simulink model "gm_sampleModel1630_sub"  (R2023a)
settings: Solver=VariableStepAuto  StartTime=0.0  StopTime=10.0  RelTol=1e-3
settings Model: Creator=user1  LastModifiedBy=user1
settings OptimizationCC: BlockReduction=off  ConditionallyExecuteInputs=off
settings DebuggingCC: InheritedTsInSrcMsg=none

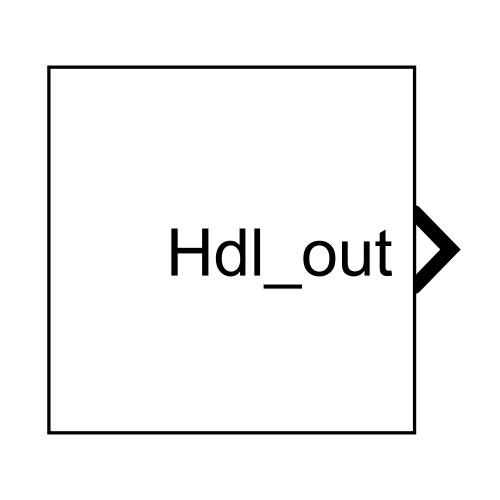
[thumbnail: Simulink's stored preview of the top-level diagram]
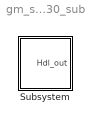
== system gm_sampleModel1630_sub ==
  Subsystem : Subsystem

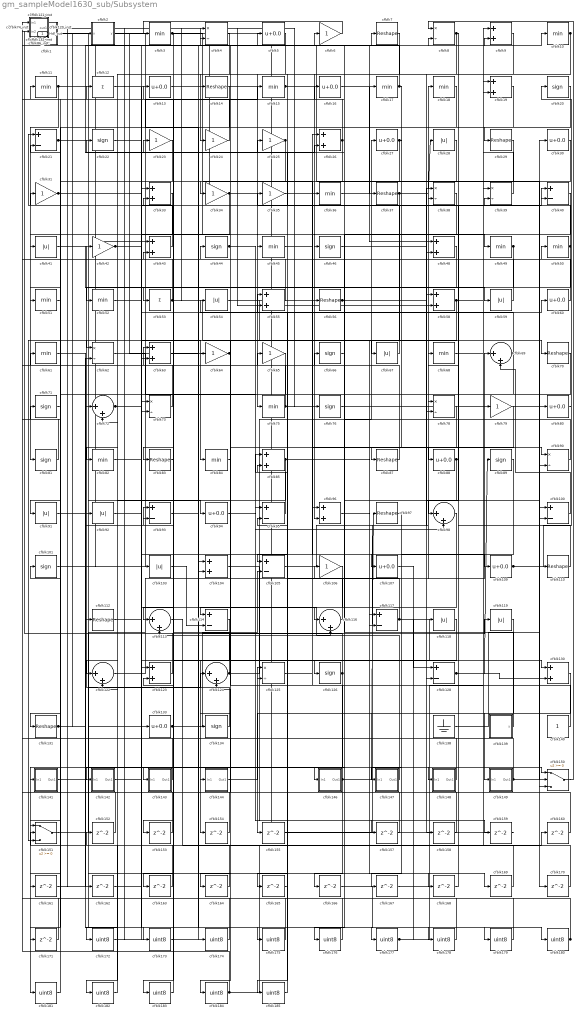
== system gm_sampleModel1630_sub/Subsystem ==
  cfblk1 : Subsystem  mask(Compare To Zero){relop=<=, OutDataTypeStr=uint8, ZeroCross=on}
      mask prompts: relop "Simulink:masks:Operator_MP"; OutDataTypeStr "Simulink:masks:OutputDataType_MP"; ZeroCross "Simulink:masks:EnableZerocrossingDetection_MP"
      mask help: Simulink:masks:CompareToZero_MD
      mask init:
      | OutDataTypeStr = 'uint8';
      | ZeroCross = 'on';
      | blkName = 'sampleModel1630_sub/Subsystem/cfblk1';
      | relop = '<=';
      | setValue = 'fixdt(0, 8)';
      mask TypeOptions relop: == | ~= | < | <= | >= | >
      mask TypeOptions OutDataTypeStr: Simulink:masks:uint8 | Simulink:masks:boolean
      mask Callback ZeroCross: sl('zeroCrossEnable', gcbh);
      mask Display: disp([relop,' 0'])
  cfblk{3,10..11,15,17..18,36,45,49..52,61,68,75,82,84} (17 alike) : MinMax  OutDataTypeStr=uint8
  cfblk{21,40,93,95,100,105,114,117,128} (9 alike) : Sum  Inputs=+-  OutDataTypeStr=uint8
  cfblk{20,22,44,46,66,71,76,81,89,101,126,134} (12 alike) : Signum
  cfblk102_inst : Subsystem
  cfblk{28,41,54,59,67,91..92,103,118..119} (10 alike) : Abs  OutDataTypeStr=uint8  SaturateOnIntegerOverflow=off
  cfblk{9,19,26,33,43,48,55,58,63,85,96,104,123,130} (14 alike) : Sum  OutDataTypeStr=uint8
  cfblk{6,23..25,31,34..35,42,64..65,79,106} (12 alike) : Gain  OutDataTypeStr=uint8
  cfblk{5,13,16,27,30,60,80,88,94,107,109,133} (12 alike) : Bias  Bias=0.0  SaturateOnIntegerOverflow=off
  cfblk108_inst : Subsystem
  cfblk{7,14,29,37,56,70,83,87,97,110,112,131} (12 alike) : Reshape
  cfblk111_inst : Subsystem
  cfblk{69,72,98,113,116,122,124} (7 alike) : Sum  Inputs=|++  OutDataTypeStr=uint8
  cfblk115_inst : Subsystem
  cfblk12 : Sum  Inputs=+  OutDataTypeStr=uint8
  cfblk120_inst : Subsystem
  cfblk121_inst : Subsystem
  cfblk{4,8,38..39,62,73,78,90,125} (9 alike) : Product  Inputs=*/  OutDataTypeStr=uint8  RndMeth=Zero  SaturateOnIntegerOverflow=on
  cfblk132_inst : Subsystem
  cfblk138 : Ground
  cfblk139 : Subsystem  mask(Counter Limited){uplimit=double(7), tsamp=double(-1)}
      mask prompts: uplimit "Simulink:masks:UpperLimit_MP"; tsamp "Simulink:masks:SampleTime_MP"
      mask help: Simulink:masks:CounterLimited_MD
      mask init:
      | nbits = double(8);
      | tsamp = double(-1);
      | uplimit = double(7);
  cfblk140 : Constant  OutDataTypeStr=uint8  SampleTime=-1
  cfblk141 : Subsystem
  cfblk142 : Subsystem
  cfblk143 : Subsystem
  cfblk144 : Subsystem
  cfblk146 : Subsystem
  cfblk147 : Subsystem
  cfblk148 : Subsystem
  cfblk149 : Subsystem
  cfblk150 : Switch  OutDataTypeStr=uint8  SaturateOnIntegerOverflow=off  InputSameDT=off
  cfblk151 : Switch  OutDataTypeStr=uint8  SaturateOnIntegerOverflow=off  InputSameDT=off
  cfblk{152..155,157..171} (19 alike) : Delay  SampleTime=1
  cfblk{172..185} (14 alike) : DataTypeConversion  OutDataTypeStr=uint8  SaturateOnIntegerOverflow=off  RndMeth=Floor
  cfblk2 : Subsystem  mask(Compare To Zero){relop=<=, OutDataTypeStr=uint8, ZeroCross=on}
      mask prompts: relop "Simulink:masks:Operator_MP"; OutDataTypeStr "Simulink:masks:OutputDataType_MP"; ZeroCross "Simulink:masks:EnableZerocrossingDetection_MP"
      mask help: Simulink:masks:CompareToZero_MD
      mask init:
      | OutDataTypeStr = 'uint8';
      | ZeroCross = 'on';
      | blkName = 'sampleModel1630_sub/Subsystem/cfblk2';
      | relop = '<=';
      | setValue = 'fixdt(0, 8)';
      mask TypeOptions relop: == | ~= | < | <= | >= | >
      mask TypeOptions OutDataTypeStr: Simulink:masks:uint8 | Simulink:masks:boolean
      mask Callback ZeroCross: sl('zeroCrossEnable', gcbh);
      mask Display: disp([relop,' 0'])
  cfblk53 : Sum  Inputs=+  OutDataTypeStr=uint8
  cfblk74_inst : Subsystem
  cfblk86_inst : Subsystem
  Hdl_out : Outport  OutDataTypeStr=uint8  SampleTime=1
  wires:
  cfblk1/1(y) -> cfblk173/1
  cfblk10/1 -> cfblk96/2, cfblk75/1
  cfblk100/1 -> cfblk69/2
  cfblk101/1 -> cfblk15/1
  cfblk102_inst/1(out1) -> cfblk80/1, cfblk162/1
  cfblk103/1 -> cfblk114/2
  cfblk104/1 -> cfblk159/1
  cfblk105/1 -> cfblk18/1
  cfblk106/1 -> cfblk114/1
  cfblk107/1 -> cfblk128/1
  cfblk108_inst/1(out1) -> cfblk103/1
  cfblk109/1 -> cfblk20/1, cfblk110/1
  cfblk11/1 -> cfblk94/1, cfblk81/1, cfblk133/1, cfblk169/1
  cfblk110/1 -> cfblk44/1
  cfblk111_inst/1(out1) -> cfblk174/1
  cfblk112/1 -> cfblk33/1
  cfblk113/1 -> cfblk160/1
  cfblk114/1 -> cfblk154/1
  cfblk115_inst/1(out1) -> cfblk58/2
  cfblk116/1 -> cfblk106/1
  cfblk117/1 -> cfblk55/1, cfblk170/1
  cfblk118/1 -> cfblk153/1
  cfblk119/1 -> cfblk155/1
  cfblk12/1 -> cfblk73/1
  cfblk120_inst/1(out1) -> cfblk56/1
  cfblk121_inst/1(out1) -> cfblk17/1
  cfblk122/1 -> cfblk69/1
  cfblk123/1 -> cfblk42/1
  cfblk124/1 -> cfblk92/1, cfblk27/1
  cfblk125/1 -> cfblk36/1
  cfblk126/1 -> cfblk181/1, cfblk108_inst/2(in2)
  cfblk128/1 -> cfblk89/1, cfblk130/2
  cfblk13/1 -> cfblk49/1
  cfblk130/1 -> cfblk149/1(In1)
  cfblk131/1 -> cfblk62/2, cfblk2/1(u)
  cfblk132_inst/1(out1) -> cfblk37/1
  cfblk133/1 -> cfblk119/1, cfblk105/2
  cfblk134/1 -> cfblk112/1
  cfblk138/1 -> cfblk100/1
  cfblk139/1(y) -> cfblk22/1
  cfblk14/1 -> cfblk163/1
  cfblk140/1 -> cfblk120_inst/2(in2)
  cfblk141/1(Out1) -> cfblk78/1
  cfblk142/1(Out1) -> cfblk123/1
  cfblk143/1(Out1) -> cfblk108_inst/1(in1)
  cfblk144/1(Out1) -> cfblk125/1
  cfblk146/1(Out1) -> cfblk97/1, cfblk96/1, cfblk166/1
  cfblk147/1(Out1) -> cfblk113/2
  cfblk148/1(Out1) -> cfblk31/1
  cfblk149/1(Out1) -> cfblk30/1, cfblk102_inst/2(in2)
  cfblk15/1 -> cfblk150/2, cfblk8/2
  cfblk150/1 -> cfblk8/1
  cfblk151/1 -> cfblk124/1
  cfblk152/1 -> cfblk121_inst/2(in2)
  cfblk153/1 -> cfblk132_inst/2(in2)
  cfblk154/1 -> cfblk115_inst/1(in1)
  cfblk155/1 -> cfblk58/1
  cfblk157/1 -> cfblk95/2
  cfblk158/1 -> cfblk124/2
  cfblk159/1 -> cfblk1/1(u)
  cfblk16/1 -> cfblk48/1
  cfblk160/1 -> cfblk33/2
  cfblk161/1 -> cfblk72/1
  cfblk162/1 -> cfblk39/2
  cfblk163/1 -> cfblk21/2
  cfblk164/1 -> cfblk123/2
  cfblk165/1 -> cfblk85/2
  cfblk166/1 -> cfblk179/1
  cfblk167/1 -> cfblk19/1
  cfblk168/1 -> cfblk38/2
  cfblk169/1 -> cfblk43/2
  cfblk17/1 -> cfblk87/1, cfblk74_inst/2(in2)
  cfblk170/1 -> cfblk151/2
  cfblk171/1 -> cfblk86_inst/2(in2)
  cfblk172/1 -> cfblk60/1
  cfblk173/1 -> cfblk7/1
  cfblk174/1 -> cfblk101/1
  cfblk175/1 -> cfblk111_inst/1(in1)
  cfblk176/1 -> cfblk111_inst/2(in2)
  cfblk177/1 -> cfblk19/2, cfblk118/1
  cfblk178/1 -> cfblk93/1
  cfblk179/1 -> cfblk93/2
  cfblk18/1 -> cfblk52/1
  cfblk180/1 -> cfblk71/1, cfblk125/2
  cfblk181/1 -> cfblk61/1
  cfblk182/1 -> cfblk152/1
  cfblk183/1 -> cfblk23/1
  cfblk184/1 -> cfblk74_inst/1(in1), cfblk79/1
  cfblk185/1 -> cfblk65/1
  cfblk19/1 -> cfblk29/1
  cfblk2/1(y) -> cfblk104/1
  cfblk20/1 -> cfblk91/1
  cfblk21/1 -> cfblk9/2, cfblk5/1, cfblk26/2
  cfblk22/1 -> cfblk46/1
  cfblk23/1 -> cfblk182/1
  cfblk24/1 -> cfblk115_inst/2(in2)
  cfblk25/1 -> cfblk131/1, cfblk62/1
  cfblk26/1 -> cfblk41/1, cfblk12/1
  cfblk27/1 -> cfblk67/1, cfblk143/1(In1)
  cfblk28/1 -> cfblk53/1
  cfblk29/1 -> cfblk34/1
  cfblk3/1 -> cfblk76/1, cfblk113/1
  cfblk30/1 -> cfblk161/1
  cfblk31/1 -> cfblk130/1, cfblk45/1
  cfblk33/1 -> cfblk51/1
  cfblk34/1 -> cfblk151/1, cfblk82/1
  cfblk35/1 -> cfblk90/1
  cfblk36/1 -> cfblk10/1
  cfblk37/1 -> cfblk28/1, cfblk100/2, cfblk84/1
  cfblk38/1 -> cfblk146/1(In1)
  cfblk39/1 -> cfblk9/1
  cfblk4/1 -> cfblk83/1
  cfblk40/1 -> cfblk48/2
  cfblk41/1 -> cfblk59/1
  cfblk42/1 -> cfblk109/1, cfblk64/1
  cfblk43/1 -> cfblk21/1
  cfblk44/1 -> cfblk98/2, cfblk150/1
  cfblk45/1 -> cfblk107/1
  cfblk46/1 -> cfblk40/1
  cfblk48/1 -> cfblk122/1
  cfblk49/1 -> cfblk122/2, cfblk73/2
  cfblk5/1 -> cfblk24/1
  cfblk50/1 -> cfblk98/1, cfblk78/2, cfblk35/1
  cfblk51/1 -> cfblk11/1
  cfblk52/1 -> cfblk4/1
  cfblk53/1 -> cfblk86_inst/1(in1), cfblk150/3
  cfblk54/1 -> cfblk117/1
  cfblk55/1 -> cfblk13/1
  cfblk56/1 -> cfblk16/1, cfblk158/1
  cfblk58/1 -> cfblk72/2, cfblk40/2, cfblk151/3, cfblk105/1, cfblk144/1(In1)
  cfblk59/1 -> cfblk39/1
  cfblk6/1 -> cfblk3/1
  cfblk60/1 -> cfblk121_inst/1(in1)
  cfblk61/1 -> cfblk180/1
  cfblk62/1 -> cfblk95/1
  cfblk63/1 -> cfblk175/1
  cfblk64/1 -> cfblk134/1, Hdl_out/1
  cfblk65/1 -> cfblk184/1
  cfblk66/1 -> cfblk6/1
  cfblk67/1 -> cfblk25/1
  cfblk68/1 -> cfblk70/1
  cfblk69/1 -> cfblk26/1, cfblk104/2, cfblk4/2
  cfblk7/1 -> cfblk172/1
  cfblk70/1 -> cfblk141/1(In1)
  cfblk71/1 -> cfblk171/1
  cfblk72/1 -> cfblk55/2, cfblk178/1, cfblk116/2
  cfblk73/1 -> cfblk63/1
  cfblk74_inst/1(out1) -> cfblk14/1
  cfblk75/1 -> cfblk102_inst/1(in1), cfblk90/2
  cfblk76/1 -> cfblk38/1
  cfblk78/1 -> cfblk164/1
  cfblk79/1 -> cfblk176/1
  cfblk8/1 -> cfblk88/1, cfblk165/1
  cfblk80/1 -> cfblk50/1
  cfblk81/1 -> cfblk120_inst/1(in1)
  cfblk82/1 -> cfblk126/1
  cfblk83/1 -> cfblk183/1
  cfblk84/1 -> cfblk54/1
  cfblk85/1 -> cfblk117/2, cfblk142/1(In1)
  cfblk86_inst/1(out1) -> cfblk43/1
  cfblk87/1 -> cfblk132_inst/1(in1)
  cfblk88/1 -> cfblk116/1, cfblk68/1
  cfblk89/1 -> cfblk147/1(In1)
  cfblk9/1 -> cfblk128/2
  cfblk90/1 -> cfblk66/1
  cfblk91/1 -> cfblk148/1(In1)
  cfblk92/1 -> cfblk63/2
  cfblk93/1 -> cfblk177/1
  cfblk94/1 -> cfblk157/1
  cfblk95/1 -> cfblk85/1
  cfblk96/1 -> cfblk168/1
  cfblk97/1 -> cfblk167/1
  cfblk98/1 -> cfblk185/1

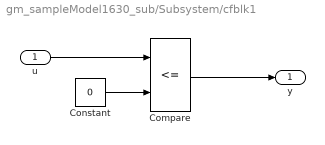
== system gm_sampleModel1630_sub/Subsystem/cfblk1 ==
  u : Inport  OutDataTypeStr=uint8  SampleTime=1
  Compare : RelationalOperator  Operator=<=  OutDataTypeStr=fixdt(0, 8)
  Constant : Constant  DisableCoverage=on  Value=0  OutDataTypeStr=Inherit: Inherit via back propagation  SampleTime=-1  PreserveConstantTs=on
  y : Outport  SampleTime=1
  wires:
  u/1 -> Compare/1
  Compare/1 -> y/1
  Constant/1 -> Compare/2

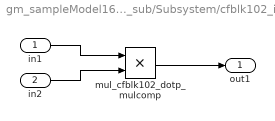
== system gm_sampleModel1630_sub/Subsystem/cfblk102_inst ==
  in1 : Inport  OutDataTypeStr=uint8  SampleTime=1
  in2 : Inport  Port=2  OutDataTypeStr=uint8  SampleTime=1
  mul_cfblk102_dotp_mulcomp : Product  Inputs=**  OutDataTypeStr=uint8  SampleTime=1
  out1 : Outport  OutDataTypeStr=uint8  SampleTime=1
  wires:
  in1/1 -> mul_cfblk102_dotp_mulcomp/1
  in2/1 -> mul_cfblk102_dotp_mulcomp/2
  mul_cfblk102_dotp_mulcomp/1 -> out1/1

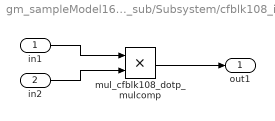
== system gm_sampleModel1630_sub/Subsystem/cfblk108_inst ==
  in1 : Inport  OutDataTypeStr=uint8  SampleTime=1
  in2 : Inport  Port=2  OutDataTypeStr=uint8  SampleTime=1
  mul_cfblk108_dotp_mulcomp : Product  Inputs=**  OutDataTypeStr=uint8  SampleTime=1
  out1 : Outport  OutDataTypeStr=uint8  SampleTime=1
  wires:
  in1/1 -> mul_cfblk108_dotp_mulcomp/1
  in2/1 -> mul_cfblk108_dotp_mulcomp/2
  mul_cfblk108_dotp_mulcomp/1 -> out1/1

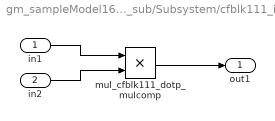
== system gm_sampleModel1630_sub/Subsystem/cfblk111_inst ==
  in1 : Inport  OutDataTypeStr=uint8  SampleTime=1
  in2 : Inport  Port=2  OutDataTypeStr=uint8  SampleTime=1
  mul_cfblk111_dotp_mulcomp : Product  Inputs=**  OutDataTypeStr=uint8  SampleTime=1
  out1 : Outport  OutDataTypeStr=uint8  SampleTime=1
  wires:
  in1/1 -> mul_cfblk111_dotp_mulcomp/1
  in2/1 -> mul_cfblk111_dotp_mulcomp/2
  mul_cfblk111_dotp_mulcomp/1 -> out1/1

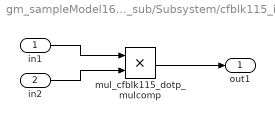
== system gm_sampleModel1630_sub/Subsystem/cfblk115_inst ==
  in1 : Inport  OutDataTypeStr=uint8  SampleTime=1
  in2 : Inport  Port=2  OutDataTypeStr=uint8  SampleTime=1
  mul_cfblk115_dotp_mulcomp : Product  Inputs=**  OutDataTypeStr=uint8  SampleTime=1
  out1 : Outport  OutDataTypeStr=uint8  SampleTime=1
  wires:
  in1/1 -> mul_cfblk115_dotp_mulcomp/1
  in2/1 -> mul_cfblk115_dotp_mulcomp/2
  mul_cfblk115_dotp_mulcomp/1 -> out1/1

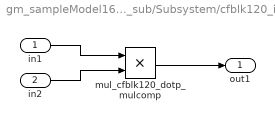
== system gm_sampleModel1630_sub/Subsystem/cfblk120_inst ==
  in1 : Inport  OutDataTypeStr=uint8  SampleTime=1
  in2 : Inport  Port=2  OutDataTypeStr=uint8  SampleTime=1
  mul_cfblk120_dotp_mulcomp : Product  Inputs=**  OutDataTypeStr=uint8  SampleTime=1
  out1 : Outport  OutDataTypeStr=uint8  SampleTime=1
  wires:
  in1/1 -> mul_cfblk120_dotp_mulcomp/1
  in2/1 -> mul_cfblk120_dotp_mulcomp/2
  mul_cfblk120_dotp_mulcomp/1 -> out1/1

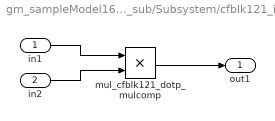
== system gm_sampleModel1630_sub/Subsystem/cfblk121_inst ==
  in1 : Inport  OutDataTypeStr=uint8  SampleTime=1
  in2 : Inport  Port=2  OutDataTypeStr=uint8  SampleTime=1
  mul_cfblk121_dotp_mulcomp : Product  Inputs=**  OutDataTypeStr=uint8  SampleTime=1
  out1 : Outport  OutDataTypeStr=uint8  SampleTime=1
  wires:
  in1/1 -> mul_cfblk121_dotp_mulcomp/1
  in2/1 -> mul_cfblk121_dotp_mulcomp/2
  mul_cfblk121_dotp_mulcomp/1 -> out1/1

== system gm_sampleModel1630_sub/Subsystem/cfblk132_inst ==
  in1 : Inport  OutDataTypeStr=uint8  SampleTime=1
  in2 : Inport  Port=2  OutDataTypeStr=uint8  SampleTime=1
  mul_cfblk132_dotp_mulcomp : Product  Inputs=**  OutDataTypeStr=uint8  SampleTime=1
  out1 : Outport  OutDataTypeStr=uint8  SampleTime=1
  wires:
  in1/1 -> mul_cfblk132_dotp_mulcomp/1
  in2/1 -> mul_cfblk132_dotp_mulcomp/2
  mul_cfblk132_dotp_mulcomp/1 -> out1/1

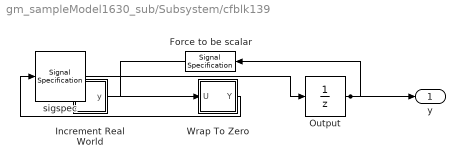
== system gm_sampleModel1630_sub/Subsystem/cfblk139 ==
  Force to be scalar : SignalSpecification  DisableCoverage=on  Dimensions=1
  Increment Real World : Subsystem  mask(Real World Value Increment){}
      mask help: Simulink:masks:RealWorldValueIncrement_MD
      mask Display: disp('V++')
  Output : UnitDelay  InitialCondition=0.0  SampleTime=tsamp  HasFrameUpgradeWarning=on
  Wrap To Zero : Subsystem  mask(Wrap To Zero){Threshold=double(7)}
      mask prompts: Threshold "Simulink:masks:Threshold_MP"
      mask help: Simulink:masks:WrapToZero_MD
  sigspec : SignalSpecification  OutDataTypeStr=uint8  Dimensions=1
  y : Outport  SampleTime=1
  wires:
  Force to be scalar/1 -> Increment Real World/1(u)
  Increment Real World/1(y) -> Wrap To Zero/1(U)
  Output/1 -> Force to be scalar/1, y/1
  Wrap To Zero/1(Y) -> sigspec/1
  sigspec/1 -> Output/1

== system gm_sampleModel1630_sub/Subsystem/cfblk141 ==
  In1 : Inport  OutDataTypeStr=uint8  PortDimensions=1  SampleTime=1
  Out1 : Outport  SampleTime=1
  wires:
  In1/1 -> Out1/1

== system gm_sampleModel1630_sub/Subsystem/cfblk142 ==
  In1 : Inport  OutDataTypeStr=uint8  PortDimensions=1  SampleTime=1
  Out1 : Outport  SampleTime=1
  wires:
  In1/1 -> Out1/1

== system gm_sampleModel1630_sub/Subsystem/cfblk143 ==
  In1 : Inport  OutDataTypeStr=uint8  PortDimensions=1  SampleTime=1
  Out1 : Outport  SampleTime=1
  wires:
  In1/1 -> Out1/1

== system gm_sampleModel1630_sub/Subsystem/cfblk144 ==
  In1 : Inport  OutDataTypeStr=uint8  PortDimensions=1  SampleTime=1
  Out1 : Outport  SampleTime=1
  wires:
  In1/1 -> Out1/1

== system gm_sampleModel1630_sub/Subsystem/cfblk146 ==
  In1 : Inport  OutDataTypeStr=uint8  PortDimensions=1  SampleTime=1
  Out1 : Outport  SampleTime=1
  wires:
  In1/1 -> Out1/1

== system gm_sampleModel1630_sub/Subsystem/cfblk147 ==
  In1 : Inport  OutDataTypeStr=uint8  PortDimensions=1  SampleTime=1
  Out1 : Outport  SampleTime=1
  wires:
  In1/1 -> Out1/1

== system gm_sampleModel1630_sub/Subsystem/cfblk148 ==
  In1 : Inport  OutDataTypeStr=uint8  PortDimensions=1  SampleTime=1
  Out1 : Outport  SampleTime=1
  wires:
  In1/1 -> Out1/1

== system gm_sampleModel1630_sub/Subsystem/cfblk149 ==
  In1 : Inport  OutDataTypeStr=uint8  PortDimensions=1  SampleTime=1
  Out1 : Outport  SampleTime=1
  wires:
  In1/1 -> Out1/1

== system gm_sampleModel1630_sub/Subsystem/cfblk2 ==
  u : Inport  OutDataTypeStr=uint8  SampleTime=1
  Compare : RelationalOperator  Operator=<=  OutDataTypeStr=fixdt(0, 8)
  Constant : Constant  DisableCoverage=on  Value=0  OutDataTypeStr=Inherit: Inherit via back propagation  SampleTime=-1  PreserveConstantTs=on
  y : Outport  SampleTime=1
  wires:
  u/1 -> Compare/1
  Compare/1 -> y/1
  Constant/1 -> Compare/2

== system gm_sampleModel1630_sub/Subsystem/cfblk74_inst ==
  in1 : Inport  OutDataTypeStr=uint8  SampleTime=1
  in2 : Inport  Port=2  OutDataTypeStr=uint8  SampleTime=1
  mul_cfblk74_dotp_mulcomp : Product  Inputs=**  OutDataTypeStr=uint8  SampleTime=1
  out1 : Outport  OutDataTypeStr=uint8  SampleTime=1
  wires:
  in1/1 -> mul_cfblk74_dotp_mulcomp/1
  in2/1 -> mul_cfblk74_dotp_mulcomp/2
  mul_cfblk74_dotp_mulcomp/1 -> out1/1

== system gm_sampleModel1630_sub/Subsystem/cfblk86_inst ==
  in1 : Inport  OutDataTypeStr=uint8  SampleTime=1
  in2 : Inport  Port=2  OutDataTypeStr=uint8  SampleTime=1
  mul_cfblk86_dotp_mulcomp : Product  Inputs=**  OutDataTypeStr=uint8  SampleTime=1
  out1 : Outport  OutDataTypeStr=uint8  SampleTime=1
  wires:
  in1/1 -> mul_cfblk86_dotp_mulcomp/1
  in2/1 -> mul_cfblk86_dotp_mulcomp/2
  mul_cfblk86_dotp_mulcomp/1 -> out1/1

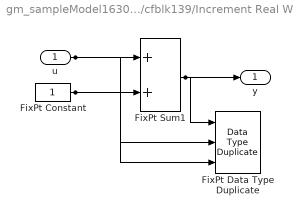
== system gm_sampleModel1630_sub/Subsystem/cfblk139/Increment Real World ==
  u : Inport  OutDataTypeStr=uint8  SampleTime=1
  FixPt Constant : Constant  DisableCoverage=on  OutDataTypeStr=Inherit: Inherit via back propagation  SampleTime=-1
  FixPt Data Type Duplicate : DataTypeDuplicate  DisableCoverage=on  NumInputPorts=3
  FixPt Sum1 : Sum  InputSameDT=on  OutDataTypeStr=Inherit: Inherit via back propagation  LockScale=on
  y : Outport  SampleTime=1
  wires:
  u/1 -> FixPt Sum1/1, FixPt Data Type Duplicate/2
  FixPt Constant/1 -> FixPt Sum1/2, FixPt Data Type Duplicate/3
  FixPt Sum1/1 -> FixPt Data Type Duplicate/1, y/1

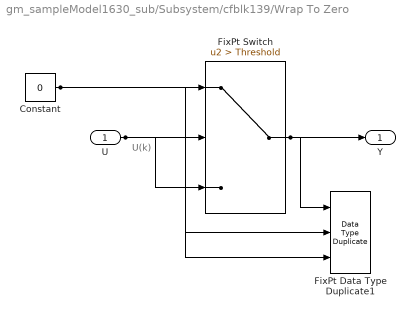
== system gm_sampleModel1630_sub/Subsystem/cfblk139/Wrap To Zero ==
  note: U(k)
  U : Inport  OutDataTypeStr=uint8  SampleTime=1
  Constant : Constant  DisableCoverage=on  Value=0  OutDataTypeStr=Inherit: Inherit via back propagation  SampleTime=-1
  FixPt Data Type Duplicate1 : DataTypeDuplicate  DisableCoverage=on  NumInputPorts=3
  FixPt Switch : Switch  Criteria=u2 > Threshold  Threshold=Threshold  OutDataTypeStr=Inherit: Inherit via back propagation  ZeroCross=off  SaturateOnIntegerOverflow=off  InputSameDT=off
  Y : Outport  SampleTime=1
  wires:
  U/1 -> FixPt Switch/3, FixPt Switch/2, FixPt Data Type Duplicate1/2
  Constant/1 -> FixPt Switch/1, FixPt Data Type Duplicate1/3
  FixPt Switch/1 -> FixPt Data Type Duplicate1/1, Y/1
